simulink model "ClosedBoxLS_model"  (R2021a)
settings: Solver=VariableStepAuto  StartTime=0.0  StopTime=tf  RelTol=1e-3
values from neighbouring files (symbols this model uses):
  a0 = Sd*(muC - 1)/Cmc    (= -11.179289014)    [ClosedBoxLS_main.m]
  a1 = Sd*(muR - 1)*Rms    (= 0.0645065691752)    [ClosedBoxLS_main.m]
  a2 = Sd*(muM - 1)*Mms    (= 0)    [ClosedBoxLS_main.m]
  b0 = Bl*muC/Cmc    (= 5799.78151854)    [ClosedBoxLS_main.m]
  b1 = Bl*muR*Rms    (= 37.6058140834)    [ClosedBoxLS_main.m]
  b2 = Bl*muM*Mms    (= 0.0897)    [ClosedBoxLS_main.m]
  Bl = 6.9    [ClosedBoxLS_main.m]
  Cmc = (1/Cms + Sd^2/Cab)^-1    (= 0.000594849993741)    [ClosedBoxLS_main.m]
  Mms = 13E-3    (= 0.013)    [ClosedBoxLS_main.m]
  Rms = 0.6    [ClosedBoxLS_main.m]
  Sd = 133E-4    (= 0.0133)    [ClosedBoxLS_main.m]
  ts = 1/fs    (= 0.0001)    [ClosedBoxLS_main.m]
undefined symbols (not defined in the file or in its folder): tau
libraries: simulink x1
settings Model: Creator=padlewsk  LastModifiedBy=padlewsk
settings DataIOCC: ReturnWorkspaceOutputs=off

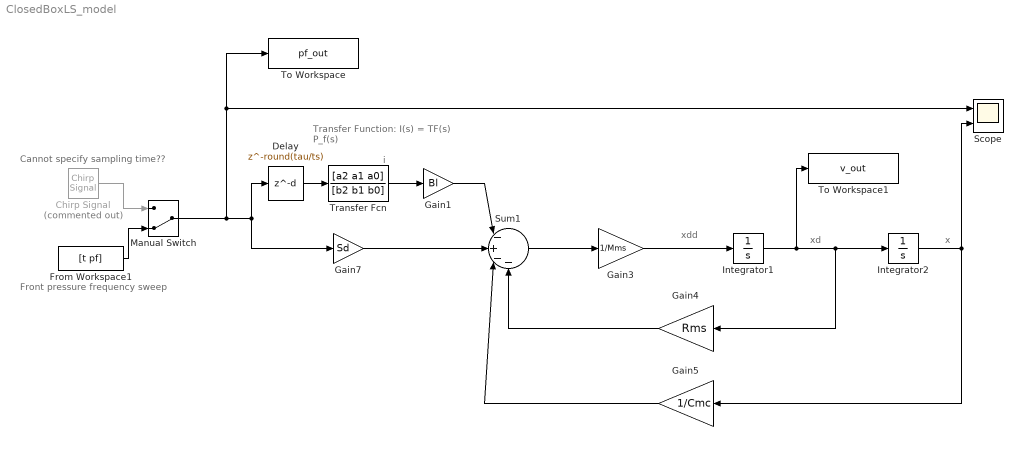
== system ClosedBoxLS_model ==
  note: Front pressure frequency sweep
  note: xd
  note: xdd
  note: x
  note: i
  note: Transfer Function:
      |   I(s) = TF(s) P_f(s)
  note: Cannot specify sampling time??
  Chirp Signal : simulink/Sources/Chirp Signal  Commented=on  f1=fi  T=tf  f2=ff
  Delay : Delay  DelayLength=round(tau/ts)
  From Workspace1 : FromWorkspace  VariableName=[t pf]  SampleTime=ts
  Gain1 : Gain  Gain=Bl
  Gain3 : Gain  Gain=1/Mms
  Gain4 : Gain  Gain=Rms
  Gain5 : Gain  Gain=1/Cmc
  Gain7 : Gain  Gain=Sd
  Integrator1 : Integrator
  Integrator2 : Integrator
  Manual Switch : ManualSwitch  CurrentSetting=0
  Scope : Scope  NumInputPorts=2
  Sum1 : Sum  Inputs=|-+--
  To Workspace : ToWorkspace  VariableName=pf_out  SaveFormat=Timeseries  SampleTime=-1
  To Workspace1 : ToWorkspace  VariableName=v_out  SaveFormat=Timeseries  SampleTime=-1
  Transfer Fcn : TransferFcn  Numerator=[a2 a1 a0]  Denominator=[b2 b1 b0]
  wires:
  Gain1/1 -> Sum1/1
  Integrator2/1 -> Scope/2, Gain5/1
  Sum1/1 -> Gain3/1
  Gain3/1 -> Integrator1/1
  Gain4/1 -> Sum1/4
  Gain5/1 -> Sum1/3
  Gain7/1 -> Sum1/2
  Transfer Fcn/1 -> Gain1/1
  Chirp Signal/1 -> Manual Switch/1
  From Workspace1/1 -> Manual Switch/2
  Manual Switch/1 -> To Workspace/1, Scope/1, Delay/1, Gain7/1
  Integrator1/1 -> To Workspace1/1, Integrator2/1, Gain4/1
  Delay/1 -> Transfer Fcn/1
